simulink model "gm_sobelFilter2024a"  (R2024a)
settings: Solver=FixedStepDiscrete  StartTime=0.0  StopTime=2  FixedStep=1/(R*C)  RelTol=1e-3
undefined symbols (not defined in the file or in its folder): gray, R
libraries: hdlsllib x5, visionhdlio x4, visionsources x2, hdlmdlgenlib x1
(part 2 of 2)

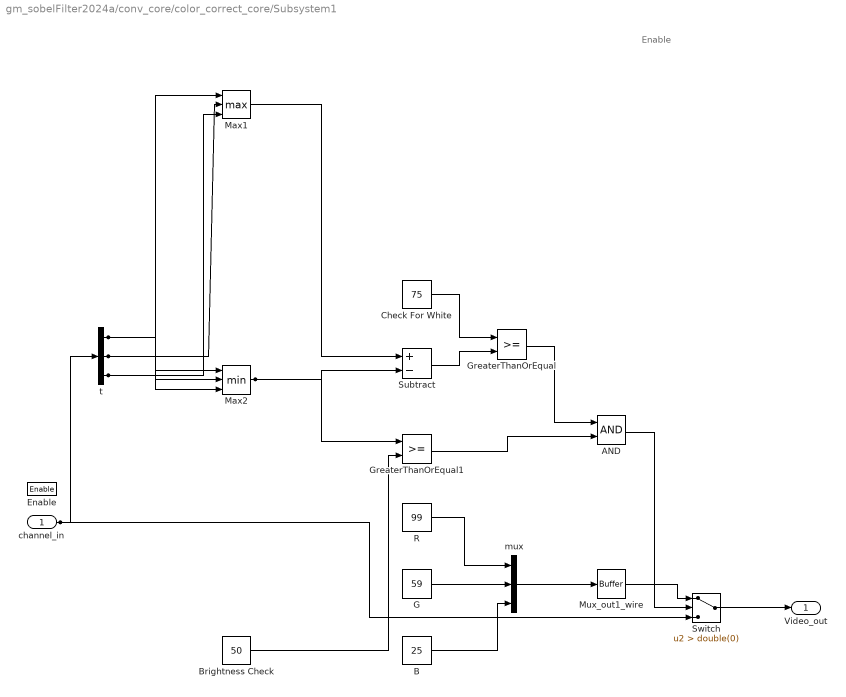
== system gm_sobelFilter2024a/conv_core/color_correct_core/Subsystem1 ==
  note: Enable
  channel_in : Inport  OutDataTypeStr=uint8  PortDimensions=[1 3]  SampleTime=2.77039007092199e-06
  Enable : EnablePort  OutDataTypeStr=boolean
  AND : Logic  AllPortsSameDT=off  OutDataTypeStr=boolean  SampleTime=2.77039007092199e-06
  B : Constant  Value=25  OutDataTypeStr=uint8  SampleTime=2.77039007092199e-06
  Brightness Check : Constant  Value=50  OutDataTypeStr=uint8  SampleTime=2.77039007092199e-06
  Check For White : Constant  Value=75  OutDataTypeStr=uint8  SampleTime=2.77039007092199e-06
  G : Constant  Value=59  OutDataTypeStr=uint8  SampleTime=2.77039007092199e-06
  GreaterThanOrEqual : RelationalOperator  OutDataTypeStr=boolean  SampleTime=2.77039007092199e-06  InputSameDT=off
  GreaterThanOrEqual1 : RelationalOperator  OutDataTypeStr=boolean  SampleTime=2.77039007092199e-06  InputSameDT=off
  Max1 : MinMax  Function=max  Inputs=3  OutDataTypeStr=uint8
  Max2 : MinMax  Inputs=3  OutDataTypeStr=uint8
  Mux_out1_wire : hdlmdlgenlib/Buffer
  R : Constant  Value=99  OutDataTypeStr=uint8  SampleTime=2.77039007092199e-06
  Subtract : Sum  Inputs=+-  OutDataTypeStr=fixdt(1, 9, 0)  AccumDataTypeStr=fixdt(1, 9, 0)  SampleTime=2.77039007092199e-06
  Switch : Switch  Criteria=u2 > Threshold  Threshold=double(0)  OutDataTypeStr=uint8  SampleTime=2.77039007092199e-06  SaturateOnIntegerOverflow=off  InputSameDT=off
  mux : Mux  Inputs=3
  t : Demux  Outputs=3
  Video_out : Outport  OutDataTypeStr=uint8  SampleTime=2.77039007092199e-06  InitialOutput=0
  wires:
  channel_in/1 -> Switch/3, t/1
  AND/1 -> Switch/2
  B/1 -> mux/3
  Brightness Check/1 -> GreaterThanOrEqual1/2
  Check For White/1 -> GreaterThanOrEqual/1
  G/1 -> mux/2
  GreaterThanOrEqual/1 -> AND/1
  GreaterThanOrEqual1/1 -> AND/2
  Max1/1 -> Subtract/1
  Max2/1 -> Subtract/2, GreaterThanOrEqual1/1
  mux/1 -> Mux_out1_wire/1
  R/1 -> mux/1
  Subtract/1 -> GreaterThanOrEqual/2
  Switch/1 -> Video_out/1
  t/1 -> Max1/1, Max2/1
  t/2 -> Max1/2, Max2/2
  t/3 -> Max1/3, Max2/3
  Mux_out1_wire/1 -> Switch/1

== system gm_sobelFilter2024a/conv_core/gaussian_conv_core/Subsystem1 ==
  note: Enable
  note: slice out gray
  channel_in : Inport  OutDataTypeStr=uint8  PortDimensions=1  SampleTime=2.77039007092199e-06
  coeffs : Inport  Port=2  OutDataTypeStr=fixdt(1, 16, 12)  PortDimensions=[9]  SampleTime=2.77039007092199e-06
  Enable : EnablePort  OutDataTypeStr=boolean
  Delay1 : Delay  DelayLength=double(1)  InitialCondition=0
  Delay2 : Delay  DelayLength=double(1)  InitialCondition=0
  Product : Product  Inputs=**  OutDataTypeStr=fixdt(1, 24, 12)  SaturateOnIntegerOverflow=on  SampleTime=2.77039007092199e-06
  Sum of Elements : Sum  Inputs=+  OutDataTypeStr=uint8  SaturateOnIntegerOverflow=on
  mux : Mux  Inputs=9
  slicer : Subsystem
  Video_out : Outport  OutDataTypeStr=uint8  SampleTime=2.77039007092199e-06  InitialOutput=0
  wires:
  channel_in/1 -> slicer/1(channel_in)
  coeffs/1 -> Product/1
  Delay1/1 -> Sum of Elements/1
  Delay2/1 -> Video_out/1
  mux/1 -> Product/2
  Product/1 -> Delay1/1
  Sum of Elements/1 -> Delay2/1
  slicer/1(out_1) -> mux/1
  slicer/2(out_2) -> mux/2
  slicer/3(out_3) -> mux/3
  slicer/4(out_4) -> mux/4
  slicer/5(out_5) -> mux/5
  slicer/6(out_6) -> mux/6
  slicer/7(out_7) -> mux/7
  slicer/8(out_8) -> mux/8
  slicer/9(out_9) -> mux/9

== system gm_sobelFilter2024a/conv_core/just_gray_core/Subsystem1 ==
  note: Enable
  note: Grayscale = (R * 0.25) + (G * 0.5) + (B * 0.0625)
  note: slice out gray
  channel_in : Inport  OutDataTypeStr=uint8  PortDimensions=[1 3]  SampleTime=2.77039007092199e-06
  Enable : EnablePort  OutDataTypeStr=boolean
  Shift Arithmetic3 : ArithShift  BitShiftNumber=double(1)  BinPtShiftNumber=double(0)
  Shift Arithmetic4 : ArithShift  BitShiftNumber=double(2)  BinPtShiftNumber=double(0)
  Shift Arithmetic5 : ArithShift  BitShiftNumber=double(4)  BinPtShiftNumber=double(0)
  Sum_stage2 : Sum  OutDataTypeStr=fixdt(0, 9, 0)  AccumDataTypeStr=uint8  SampleTime=2.77039007092199e-06
  Sum_stage3 : Sum  OutDataTypeStr=uint8  AccumDataTypeStr=uint8  SampleTime=2.77039007092199e-06
  t : Demux  Outputs=3
  Video_out : Outport  OutDataTypeStr=uint8  SampleTime=2.77039007092199e-06  InitialOutput=0
  wires:
  channel_in/1 -> t/1
  Shift Arithmetic3/1 -> Sum_stage2/2
  Shift Arithmetic4/1 -> Sum_stage2/1
  Shift Arithmetic5/1 -> Sum_stage3/2
  Sum_stage3/1 -> Video_out/1
  t/1 -> Shift Arithmetic4/1
  t/2 -> Shift Arithmetic3/1
  t/3 -> Shift Arithmetic5/1
  Sum_stage2/1 -> Sum_stage3/1

== system gm_sobelFilter2024a/conv_core/normalize image/Subsystem1 ==
  note: Enable
  note: Normalize Image (Assuming Max is 115)
  channel_in : Inport  OutDataTypeStr=uint8  PortDimensions=1  SampleTime=2.77039007092199e-06
  Enable : EnablePort  OutDataTypeStr=boolean
  Delay2 : Delay  DelayLength=double(4)  InitialCondition=0
  GreaterThanOrEqual : RelationalOperator  OutDataTypeStr=boolean  SampleTime=2.77039007092199e-06  InputSameDT=off
  Max1 : Constant  Value=115  OutDataTypeStr=uint8  SampleTime=2.77039007092199e-06
  Max2 : Constant  Value=0  OutDataTypeStr=uint8  SampleTime=2.77039007092199e-06
  Switch1 : Switch  Criteria=u2 > Threshold  Threshold=double(0)  OutDataTypeStr=uint8  SampleTime=2.77039007092199e-06  SaturateOnIntegerOverflow=off  InputSameDT=off
  Video_out : Outport  OutDataTypeStr=uint8  SampleTime=2.77039007092199e-06  InitialOutput=0
  wires:
  channel_in/1 -> Switch1/1, GreaterThanOrEqual/1
  Delay2/1 -> Video_out/1
  GreaterThanOrEqual/1 -> Switch1/2
  Max1/1 -> GreaterThanOrEqual/2
  Max2/1 -> Switch1/3
  Switch1/1 -> Delay2/1

== system gm_sobelFilter2024a/conv_core/sobel_horz_conv_core/Subsystem1 ==
  note: Enable
  note: slice out gray
  channel_in : Inport  OutDataTypeStr=uint8  PortDimensions=1  SampleTime=2.77039007092199e-06
  coeffs : Inport  Port=2  OutDataTypeStr=fixdt(1, 16, 12)  PortDimensions=[9]  SampleTime=2.77039007092199e-06
  Enable : EnablePort  OutDataTypeStr=boolean
  Delay1 : Delay  DelayLength=double(1)  InitialCondition=0
  Delay2 : Delay  DelayLength=double(1)  InitialCondition=0
  Product : Product  Inputs=**  OutDataTypeStr=fixdt(1, 24, 12)  SaturateOnIntegerOverflow=on  SampleTime=2.77039007092199e-06
  Sum of Elements : Sum  Inputs=+  OutDataTypeStr=uint8  SaturateOnIntegerOverflow=on
  mux : Mux  Inputs=9
  slicer : Subsystem
  Video_out : Outport  OutDataTypeStr=uint8  SampleTime=2.77039007092199e-06  InitialOutput=0
  wires:
  channel_in/1 -> slicer/1(channel_in)
  coeffs/1 -> Product/1
  Delay1/1 -> Sum of Elements/1
  Delay2/1 -> Video_out/1
  mux/1 -> Product/2
  Product/1 -> Delay1/1
  Sum of Elements/1 -> Delay2/1
  slicer/1(out_1) -> mux/1
  slicer/2(out_2) -> mux/2
  slicer/3(out_3) -> mux/3
  slicer/4(out_4) -> mux/4
  slicer/5(out_5) -> mux/5
  slicer/6(out_6) -> mux/6
  slicer/7(out_7) -> mux/7
  slicer/8(out_8) -> mux/8
  slicer/9(out_9) -> mux/9

== system gm_sobelFilter2024a/conv_core/sobel_horz_conv_core_alt/Subsystem1 ==
  note: Enable
  note: slice out gray
  channel_in : Inport  OutDataTypeStr=uint8  PortDimensions=1  SampleTime=2.77039007092199e-06
  coeffs : Inport  Port=2  OutDataTypeStr=fixdt(1, 16, 12)  PortDimensions=[9]  SampleTime=2.77039007092199e-06
  Enable : EnablePort  OutDataTypeStr=boolean
  Delay1 : Delay  DelayLength=double(1)  InitialCondition=0
  Delay2 : Delay  DelayLength=double(1)  InitialCondition=0
  Product : Product  Inputs=**  OutDataTypeStr=fixdt(1, 24, 12)  SaturateOnIntegerOverflow=on  SampleTime=2.77039007092199e-06
  Sum of Elements : Sum  Inputs=+  OutDataTypeStr=uint8  SaturateOnIntegerOverflow=on
  mux : Mux  Inputs=9
  slicer : Subsystem
  Video_out : Outport  OutDataTypeStr=uint8  SampleTime=2.77039007092199e-06  InitialOutput=0
  wires:
  channel_in/1 -> slicer/1(channel_in)
  coeffs/1 -> Product/1
  Delay1/1 -> Sum of Elements/1
  Delay2/1 -> Video_out/1
  mux/1 -> Product/2
  Product/1 -> Delay1/1
  Sum of Elements/1 -> Delay2/1
  slicer/1(out_1) -> mux/1
  slicer/2(out_2) -> mux/2
  slicer/3(out_3) -> mux/3
  slicer/4(out_4) -> mux/4
  slicer/5(out_5) -> mux/5
  slicer/6(out_6) -> mux/6
  slicer/7(out_7) -> mux/7
  slicer/8(out_8) -> mux/8
  slicer/9(out_9) -> mux/9

== system gm_sobelFilter2024a/conv_core/sobel_vert_conv_core/Subsystem1 ==
  note: Enable
  note: slice out gray
  channel_in : Inport  OutDataTypeStr=uint8  PortDimensions=1  SampleTime=2.77039007092199e-06
  coeffs : Inport  Port=2  OutDataTypeStr=fixdt(1, 16, 12)  PortDimensions=[9]  SampleTime=2.77039007092199e-06
  Enable : EnablePort  OutDataTypeStr=boolean
  Delay1 : Delay  DelayLength=double(1)  InitialCondition=0
  Delay2 : Delay  DelayLength=double(1)  InitialCondition=0
  Product : Product  Inputs=**  OutDataTypeStr=fixdt(1, 24, 12)  SaturateOnIntegerOverflow=on  SampleTime=2.77039007092199e-06
  Sum of Elements : Sum  Inputs=+  OutDataTypeStr=uint8  SaturateOnIntegerOverflow=on
  mux : Mux  Inputs=9
  slicer : Subsystem
  Video_out : Outport  OutDataTypeStr=uint8  SampleTime=2.77039007092199e-06  InitialOutput=0
  wires:
  channel_in/1 -> slicer/1(channel_in)
  coeffs/1 -> Product/1
  Delay1/1 -> Sum of Elements/1
  Delay2/1 -> Video_out/1
  mux/1 -> Product/2
  Product/1 -> Delay1/1
  Sum of Elements/1 -> Delay2/1
  slicer/1(out_1) -> mux/1
  slicer/2(out_2) -> mux/2
  slicer/3(out_3) -> mux/3
  slicer/4(out_4) -> mux/4
  slicer/5(out_5) -> mux/5
  slicer/6(out_6) -> mux/6
  slicer/7(out_7) -> mux/7
  slicer/8(out_8) -> mux/8
  slicer/9(out_9) -> mux/9

== system gm_sobelFilter2024a/conv_core/sobel_vert_conv_core_alt/Subsystem1 ==
  note: Enable
  note: slice out gray
  channel_in : Inport  OutDataTypeStr=uint8  PortDimensions=1  SampleTime=2.77039007092199e-06
  coeffs : Inport  Port=2  OutDataTypeStr=fixdt(1, 16, 12)  PortDimensions=[9]  SampleTime=2.77039007092199e-06
  Enable : EnablePort  OutDataTypeStr=boolean
  Delay1 : Delay  DelayLength=double(1)  InitialCondition=0
  Delay2 : Delay  DelayLength=double(1)  InitialCondition=0
  Product : Product  Inputs=**  OutDataTypeStr=fixdt(1, 24, 12)  SaturateOnIntegerOverflow=on  SampleTime=2.77039007092199e-06
  Sum of Elements : Sum  Inputs=+  OutDataTypeStr=uint8  SaturateOnIntegerOverflow=on
  mux : Mux  Inputs=9
  slicer : Subsystem
  Video_out : Outport  OutDataTypeStr=uint8  SampleTime=2.77039007092199e-06  InitialOutput=0
  wires:
  channel_in/1 -> slicer/1(channel_in)
  coeffs/1 -> Product/1
  Delay1/1 -> Sum of Elements/1
  Delay2/1 -> Video_out/1
  mux/1 -> Product/2
  Product/1 -> Delay1/1
  Sum of Elements/1 -> Delay2/1
  slicer/1(out_1) -> mux/1
  slicer/2(out_2) -> mux/2
  slicer/3(out_3) -> mux/3
  slicer/4(out_4) -> mux/4
  slicer/5(out_5) -> mux/5
  slicer/6(out_6) -> mux/6
  slicer/7(out_7) -> mux/7
  slicer/8(out_8) -> mux/8
  slicer/9(out_9) -> mux/9

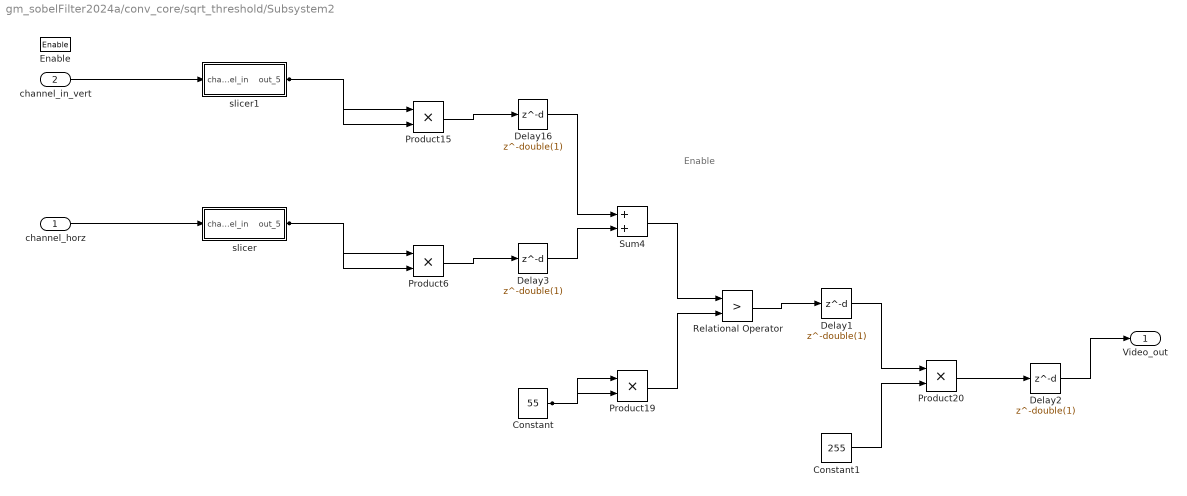
== system gm_sobelFilter2024a/conv_core/sqrt_threshold/Subsystem2 ==
  note: Enable
  channel_horz : Inport  OutDataTypeStr=uint8  PortDimensions=1  SampleTime=2.77039007092199e-06
  channel_in_vert : Inport  Port=2  OutDataTypeStr=uint8  PortDimensions=1  SampleTime=2.77039007092199e-06
  Enable : EnablePort  OutDataTypeStr=boolean
  Constant : Constant  Value=55  OutDataTypeStr=uint8  SampleTime=2.77039007092199e-06
  Constant1 : Constant  Value=255  OutDataTypeStr=uint8  SampleTime=2.77039007092199e-06
  Delay{1..3,16} (4 alike) : Delay  DelayLength=double(1)  InitialCondition=0
  Product15 : Product  Inputs=**  OutDataTypeStr=uint16  SaturateOnIntegerOverflow=on  SampleTime=2.77039007092199e-06
  Product19 : Product  Inputs=**  OutDataTypeStr=uint16  SaturateOnIntegerOverflow=on  SampleTime=2.77039007092199e-06
  Product20 : Product  Inputs=**  OutDataTypeStr=uint8  SaturateOnIntegerOverflow=on  SampleTime=2.77039007092199e-06
  Product6 : Product  Inputs=**  OutDataTypeStr=uint16  SaturateOnIntegerOverflow=on  SampleTime=2.77039007092199e-06
  Relational Operator : RelationalOperator  Operator=>  OutDataTypeStr=boolean  SampleTime=2.77039007092199e-06  InputSameDT=off
  Sum4 : Sum  OutDataTypeStr=fixdt(0, 17, 0)  AccumDataTypeStr=fixdt(0, 17, 0)  SampleTime=2.77039007092199e-06
  slicer : Subsystem
  slicer1 : Subsystem
  Video_out : Outport  OutDataTypeStr=uint8  SampleTime=2.77039007092199e-06  InitialOutput=0
  wires:
  channel_horz/1 -> slicer/1(channel_in)
  channel_in_vert/1 -> slicer1/1(channel_in)
  Constant/1 -> Product19/2, Product19/1
  Constant1/1 -> Product20/2
  Delay1/1 -> Product20/1
  Delay16/1 -> Sum4/1
  Delay2/1 -> Video_out/1
  Delay3/1 -> Sum4/2
  Product15/1 -> Delay16/1
  Product19/1 -> Relational Operator/2
  Product20/1 -> Delay2/1
  Product6/1 -> Delay3/1
  Relational Operator/1 -> Delay1/1
  Sum4/1 -> Relational Operator/1
  slicer/1(out_5) -> Product6/2, Product6/1
  slicer1/1(out_5) -> Product15/2, Product15/1

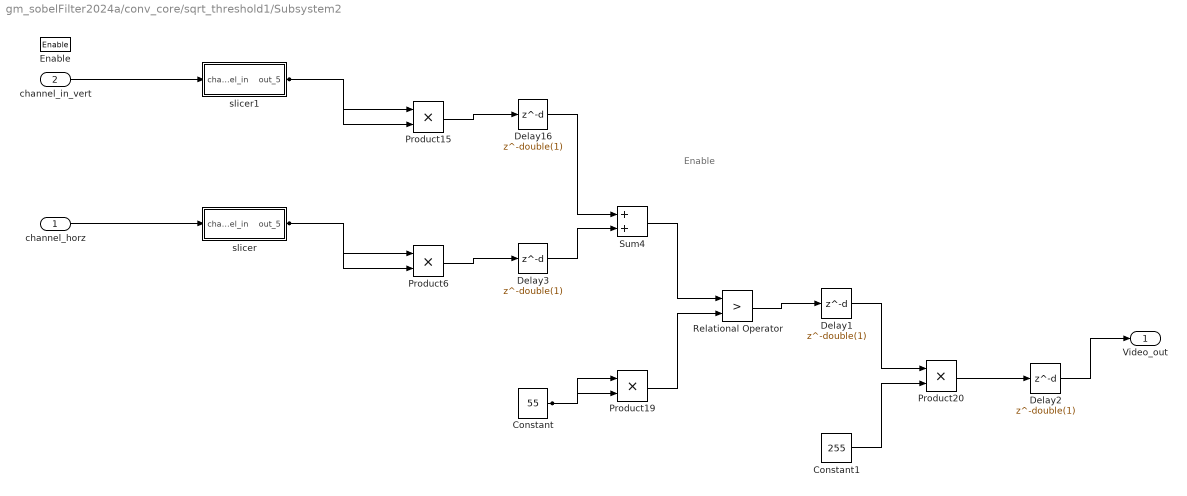
== system gm_sobelFilter2024a/conv_core/sqrt_threshold1/Subsystem2 ==
  note: Enable
  channel_horz : Inport  OutDataTypeStr=uint8  PortDimensions=1  SampleTime=2.77039007092199e-06
  channel_in_vert : Inport  Port=2  OutDataTypeStr=uint8  PortDimensions=1  SampleTime=2.77039007092199e-06
  Enable : EnablePort  OutDataTypeStr=boolean
  Constant : Constant  Value=55  OutDataTypeStr=uint8  SampleTime=2.77039007092199e-06
  Constant1 : Constant  Value=255  OutDataTypeStr=uint8  SampleTime=2.77039007092199e-06
  Delay{1..3,16} (4 alike) : Delay  DelayLength=double(1)  InitialCondition=0
  Product15 : Product  Inputs=**  OutDataTypeStr=uint16  SaturateOnIntegerOverflow=on  SampleTime=2.77039007092199e-06
  Product19 : Product  Inputs=**  OutDataTypeStr=uint16  SaturateOnIntegerOverflow=on  SampleTime=2.77039007092199e-06
  Product20 : Product  Inputs=**  OutDataTypeStr=uint8  SaturateOnIntegerOverflow=on  SampleTime=2.77039007092199e-06
  Product6 : Product  Inputs=**  OutDataTypeStr=uint16  SaturateOnIntegerOverflow=on  SampleTime=2.77039007092199e-06
  Relational Operator : RelationalOperator  Operator=>  OutDataTypeStr=boolean  SampleTime=2.77039007092199e-06  InputSameDT=off
  Sum4 : Sum  OutDataTypeStr=fixdt(0, 17, 0)  AccumDataTypeStr=fixdt(0, 17, 0)  SampleTime=2.77039007092199e-06
  slicer : Subsystem
  slicer1 : Subsystem
  Video_out : Outport  OutDataTypeStr=uint8  SampleTime=2.77039007092199e-06  InitialOutput=0
  wires:
  slicer1/1(out_5) -> Product15/1, Product15/2
  slicer/1(out_5) -> Product6/1, Product6/2
  Sum4/1 -> Relational Operator/1
  Relational Operator/1 -> Delay1/1
  Product6/1 -> Delay3/1
  Product20/1 -> Delay2/1
  Product19/1 -> Relational Operator/2
  Product15/1 -> Delay16/1
  Delay3/1 -> Sum4/2
  Delay2/1 -> Video_out/1
  Delay16/1 -> Sum4/1
  Delay1/1 -> Product20/1
  Constant1/1 -> Product20/2
  Constant/1 -> Product19/1, Product19/2
  channel_in_vert/1 -> slicer1/1(channel_in)
  channel_horz/1 -> slicer/1(channel_in)

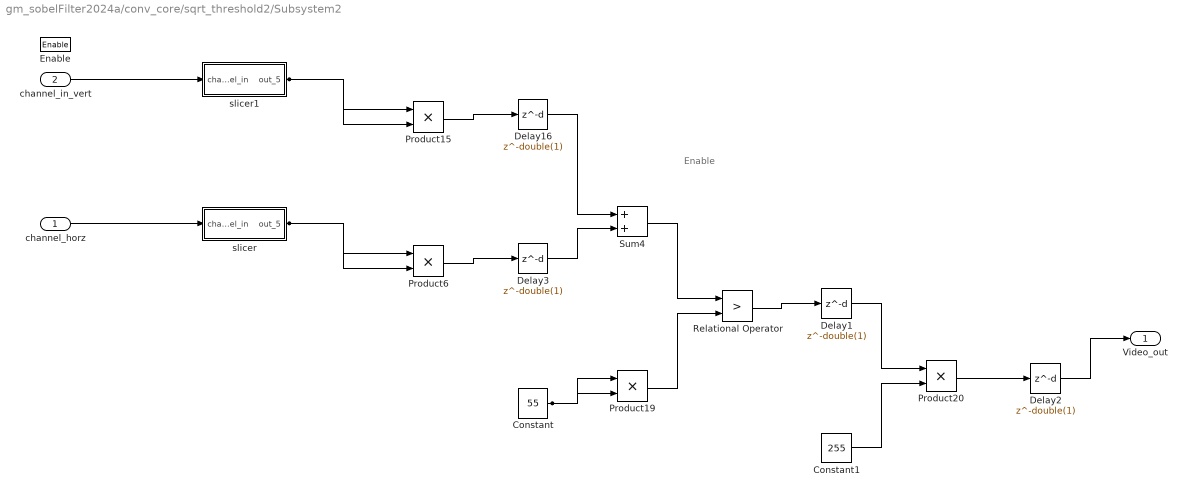
== system gm_sobelFilter2024a/conv_core/sqrt_threshold2/Subsystem2 ==
  note: Enable
  channel_horz : Inport  OutDataTypeStr=uint8  PortDimensions=1  SampleTime=2.77039007092199e-06
  channel_in_vert : Inport  Port=2  OutDataTypeStr=uint8  PortDimensions=1  SampleTime=2.77039007092199e-06
  Enable : EnablePort  OutDataTypeStr=boolean
  Constant : Constant  Value=55  OutDataTypeStr=uint8  SampleTime=2.77039007092199e-06
  Constant1 : Constant  Value=255  OutDataTypeStr=uint8  SampleTime=2.77039007092199e-06
  Delay{1..3,16} (4 alike) : Delay  DelayLength=double(1)  InitialCondition=0
  Product15 : Product  Inputs=**  OutDataTypeStr=uint16  SaturateOnIntegerOverflow=on  SampleTime=2.77039007092199e-06
  Product19 : Product  Inputs=**  OutDataTypeStr=uint16  SaturateOnIntegerOverflow=on  SampleTime=2.77039007092199e-06
  Product20 : Product  Inputs=**  OutDataTypeStr=uint8  SaturateOnIntegerOverflow=on  SampleTime=2.77039007092199e-06
  Product6 : Product  Inputs=**  OutDataTypeStr=uint16  SaturateOnIntegerOverflow=on  SampleTime=2.77039007092199e-06
  Relational Operator : RelationalOperator  Operator=>  OutDataTypeStr=boolean  SampleTime=2.77039007092199e-06  InputSameDT=off
  Sum4 : Sum  OutDataTypeStr=fixdt(0, 17, 0)  AccumDataTypeStr=fixdt(0, 17, 0)  SampleTime=2.77039007092199e-06
  slicer : Subsystem
  slicer1 : Subsystem
  Video_out : Outport  OutDataTypeStr=uint8  SampleTime=2.77039007092199e-06  InitialOutput=0
  wires:
  slicer1/1(out_5) -> Product15/1, Product15/2
  slicer/1(out_5) -> Product6/1, Product6/2
  Sum4/1 -> Relational Operator/1
  Relational Operator/1 -> Delay1/1
  Product6/1 -> Delay3/1
  Product20/1 -> Delay2/1
  Product19/1 -> Relational Operator/2
  Product15/1 -> Delay16/1
  Delay3/1 -> Sum4/2
  Delay2/1 -> Video_out/1
  Delay16/1 -> Sum4/1
  Delay1/1 -> Product20/1
  Constant1/1 -> Product20/2
  Constant/1 -> Product19/1, Product19/2
  channel_in_vert/1 -> slicer1/1(channel_in)
  channel_horz/1 -> slicer/1(channel_in)

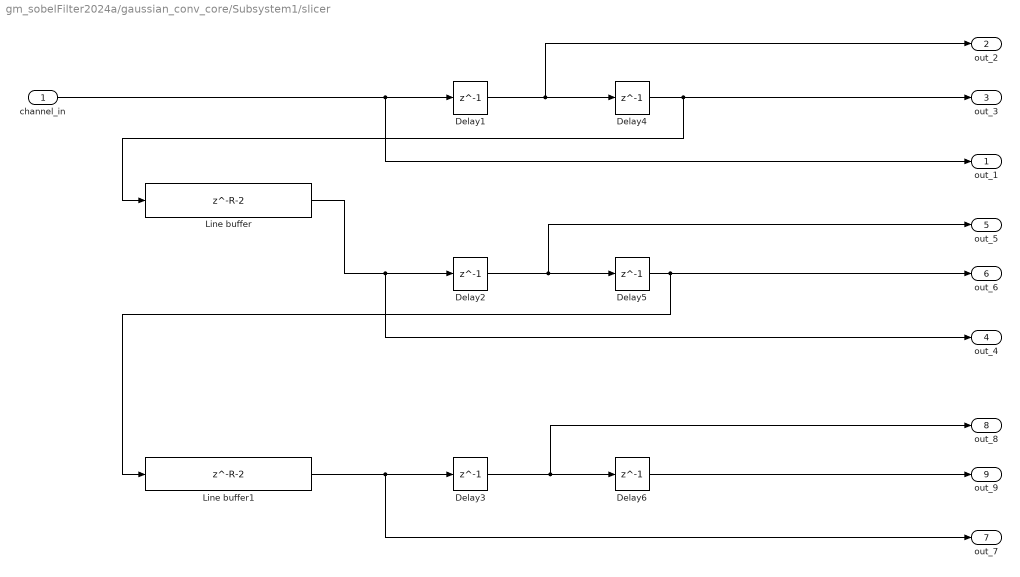
== system gm_sobelFilter2024a/gaussian_conv_core/Subsystem1/slicer ==
  channel_in : Inport
  Delay{1..6} (6 alike) : Delay  DelayLength=1  InitialCondition=0
  Line buffer : Delay  DelayLength=R-2  InitialCondition=0
  Line buffer1 : Delay  DelayLength=R-2  InitialCondition=0
  out_1 : Outport  VectorParamsAs1DForOutWhenUnconnected=off
  out_2 : Outport  Port=2  VectorParamsAs1DForOutWhenUnconnected=off
  out_3 : Outport  Port=3  VectorParamsAs1DForOutWhenUnconnected=off
  out_4 : Outport  Port=4  VectorParamsAs1DForOutWhenUnconnected=off
  out_5 : Outport  Port=5  VectorParamsAs1DForOutWhenUnconnected=off
  out_6 : Outport  Port=6  VectorParamsAs1DForOutWhenUnconnected=off
  out_7 : Outport  Port=7  VectorParamsAs1DForOutWhenUnconnected=off
  out_8 : Outport  Port=8  VectorParamsAs1DForOutWhenUnconnected=off
  out_9 : Outport  Port=9  VectorParamsAs1DForOutWhenUnconnected=off
  wires:
  Delay2/1 -> Delay5/1, out_5/1
  Line buffer1/1 -> Delay3/1, out_7/1
  Line buffer/1 -> Delay2/1, out_4/1
  Delay6/1 -> out_9/1
  Delay5/1 -> out_6/1, Line buffer1/1
  Delay3/1 -> Delay6/1, out_8/1
  Delay1/1 -> Delay4/1, out_2/1
  channel_in/1 -> Delay1/1, out_1/1
  Delay4/1 -> out_3/1, Line buffer/1

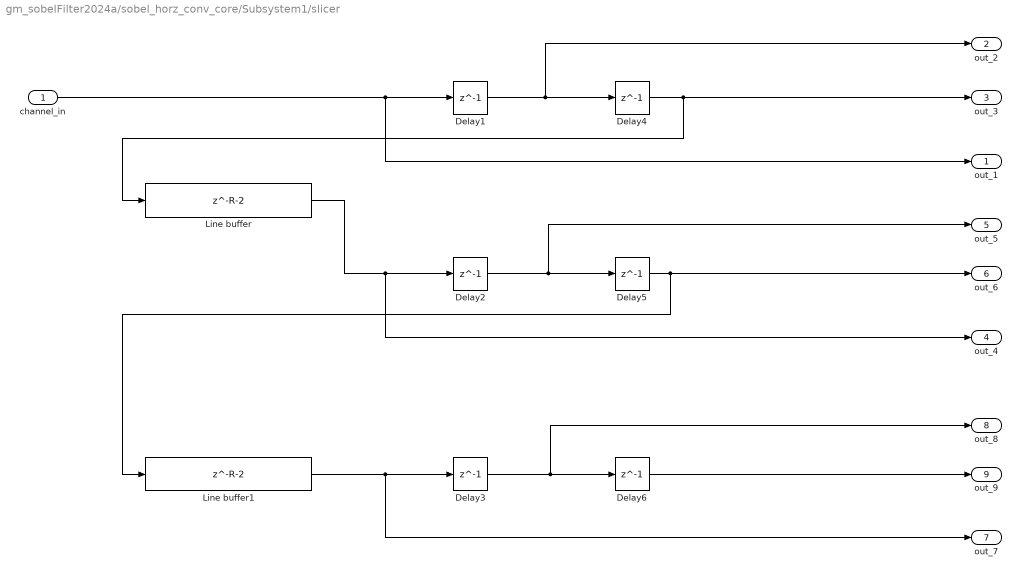
== system gm_sobelFilter2024a/sobel_horz_conv_core/Subsystem1/slicer ==
  channel_in : Inport
  Delay{1..6} (6 alike) : Delay  DelayLength=1  InitialCondition=0
  Line buffer : Delay  DelayLength=R-2  InitialCondition=0
  Line buffer1 : Delay  DelayLength=R-2  InitialCondition=0
  out_1 : Outport  VectorParamsAs1DForOutWhenUnconnected=off
  out_2 : Outport  Port=2  VectorParamsAs1DForOutWhenUnconnected=off
  out_3 : Outport  Port=3  VectorParamsAs1DForOutWhenUnconnected=off
  out_4 : Outport  Port=4  VectorParamsAs1DForOutWhenUnconnected=off
  out_5 : Outport  Port=5  VectorParamsAs1DForOutWhenUnconnected=off
  out_6 : Outport  Port=6  VectorParamsAs1DForOutWhenUnconnected=off
  out_7 : Outport  Port=7  VectorParamsAs1DForOutWhenUnconnected=off
  out_8 : Outport  Port=8  VectorParamsAs1DForOutWhenUnconnected=off
  out_9 : Outport  Port=9  VectorParamsAs1DForOutWhenUnconnected=off
  wires:
  Delay2/1 -> Delay5/1, out_5/1
  Line buffer1/1 -> Delay3/1, out_7/1
  Line buffer/1 -> Delay2/1, out_4/1
  Delay6/1 -> out_9/1
  Delay5/1 -> out_6/1, Line buffer1/1
  Delay3/1 -> Delay6/1, out_8/1
  Delay1/1 -> Delay4/1, out_2/1
  channel_in/1 -> Delay1/1, out_1/1
  Delay4/1 -> out_3/1, Line buffer/1

== system gm_sobelFilter2024a/sobel_horz_conv_core_alt/Subsystem1/slicer ==
  channel_in : Inport
  Delay{1..6} (6 alike) : Delay  DelayLength=1  InitialCondition=0
  Line buffer : Delay  DelayLength=R-2  InitialCondition=0
  Line buffer1 : Delay  DelayLength=R-2  InitialCondition=0
  out_1 : Outport  VectorParamsAs1DForOutWhenUnconnected=off
  out_2 : Outport  Port=2  VectorParamsAs1DForOutWhenUnconnected=off
  out_3 : Outport  Port=3  VectorParamsAs1DForOutWhenUnconnected=off
  out_4 : Outport  Port=4  VectorParamsAs1DForOutWhenUnconnected=off
  out_5 : Outport  Port=5  VectorParamsAs1DForOutWhenUnconnected=off
  out_6 : Outport  Port=6  VectorParamsAs1DForOutWhenUnconnected=off
  out_7 : Outport  Port=7  VectorParamsAs1DForOutWhenUnconnected=off
  out_8 : Outport  Port=8  VectorParamsAs1DForOutWhenUnconnected=off
  out_9 : Outport  Port=9  VectorParamsAs1DForOutWhenUnconnected=off
  wires:
  Delay2/1 -> Delay5/1, out_5/1
  Line buffer1/1 -> Delay3/1, out_7/1
  Line buffer/1 -> Delay2/1, out_4/1
  Delay6/1 -> out_9/1
  Delay5/1 -> out_6/1, Line buffer1/1
  Delay3/1 -> Delay6/1, out_8/1
  Delay1/1 -> Delay4/1, out_2/1
  channel_in/1 -> Delay1/1, out_1/1
  Delay4/1 -> out_3/1, Line buffer/1

== system gm_sobelFilter2024a/sobel_vert_conv_core/Subsystem1/slicer ==
  channel_in : Inport
  Delay{1..6} (6 alike) : Delay  DelayLength=1  InitialCondition=0
  Line buffer : Delay  DelayLength=R-2  InitialCondition=0
  Line buffer1 : Delay  DelayLength=R-2  InitialCondition=0
  out_1 : Outport  VectorParamsAs1DForOutWhenUnconnected=off
  out_2 : Outport  Port=2  VectorParamsAs1DForOutWhenUnconnected=off
  out_3 : Outport  Port=3  VectorParamsAs1DForOutWhenUnconnected=off
  out_4 : Outport  Port=4  VectorParamsAs1DForOutWhenUnconnected=off
  out_5 : Outport  Port=5  VectorParamsAs1DForOutWhenUnconnected=off
  out_6 : Outport  Port=6  VectorParamsAs1DForOutWhenUnconnected=off
  out_7 : Outport  Port=7  VectorParamsAs1DForOutWhenUnconnected=off
  out_8 : Outport  Port=8  VectorParamsAs1DForOutWhenUnconnected=off
  out_9 : Outport  Port=9  VectorParamsAs1DForOutWhenUnconnected=off
  wires:
  Delay2/1 -> Delay5/1, out_5/1
  Line buffer1/1 -> Delay3/1, out_7/1
  Line buffer/1 -> Delay2/1, out_4/1
  Delay6/1 -> out_9/1
  Delay5/1 -> out_6/1, Line buffer1/1
  Delay3/1 -> Delay6/1, out_8/1
  Delay1/1 -> Delay4/1, out_2/1
  channel_in/1 -> Delay1/1, out_1/1
  Delay4/1 -> out_3/1, Line buffer/1

== system gm_sobelFilter2024a/sobel_vert_conv_core_alt/Subsystem1/slicer ==
  channel_in : Inport
  Delay{1..6} (6 alike) : Delay  DelayLength=1  InitialCondition=0
  Line buffer : Delay  DelayLength=R-2  InitialCondition=0
  Line buffer1 : Delay  DelayLength=R-2  InitialCondition=0
  out_1 : Outport  VectorParamsAs1DForOutWhenUnconnected=off
  out_2 : Outport  Port=2  VectorParamsAs1DForOutWhenUnconnected=off
  out_3 : Outport  Port=3  VectorParamsAs1DForOutWhenUnconnected=off
  out_4 : Outport  Port=4  VectorParamsAs1DForOutWhenUnconnected=off
  out_5 : Outport  Port=5  VectorParamsAs1DForOutWhenUnconnected=off
  out_6 : Outport  Port=6  VectorParamsAs1DForOutWhenUnconnected=off
  out_7 : Outport  Port=7  VectorParamsAs1DForOutWhenUnconnected=off
  out_8 : Outport  Port=8  VectorParamsAs1DForOutWhenUnconnected=off
  out_9 : Outport  Port=9  VectorParamsAs1DForOutWhenUnconnected=off
  wires:
  Delay2/1 -> Delay5/1, out_5/1
  Line buffer1/1 -> Delay3/1, out_7/1
  Line buffer/1 -> Delay2/1, out_4/1
  Delay6/1 -> out_9/1
  Delay5/1 -> out_6/1, Line buffer1/1
  Delay3/1 -> Delay6/1, out_8/1
  Delay1/1 -> Delay4/1, out_2/1
  channel_in/1 -> Delay1/1, out_1/1
  Delay4/1 -> out_3/1, Line buffer/1

== system gm_sobelFilter2024a/sqrt_threshold/Subsystem2/slicer ==
  channel_in : Inport
  Delay{1..6} (6 alike) : Delay  DelayLength=1  InitialCondition=0
  Line buffer : Delay  DelayLength=R-2  InitialCondition=0
  Line buffer1 : Delay  DelayLength=R-2  InitialCondition=0
  out_1 : Outport  VectorParamsAs1DForOutWhenUnconnected=off
  out_2 : Outport  Port=2  VectorParamsAs1DForOutWhenUnconnected=off
  out_3 : Outport  Port=3  VectorParamsAs1DForOutWhenUnconnected=off
  out_4 : Outport  Port=4  VectorParamsAs1DForOutWhenUnconnected=off
  out_5 : Outport  Port=5  VectorParamsAs1DForOutWhenUnconnected=off
  out_6 : Outport  Port=6  VectorParamsAs1DForOutWhenUnconnected=off
  out_7 : Outport  Port=7  VectorParamsAs1DForOutWhenUnconnected=off
  out_8 : Outport  Port=8  VectorParamsAs1DForOutWhenUnconnected=off
  out_9 : Outport  Port=9  VectorParamsAs1DForOutWhenUnconnected=off
  wires:
  Delay2/1 -> Delay5/1, out_5/1
  Line buffer1/1 -> Delay3/1, out_7/1
  Line buffer/1 -> Delay2/1, out_4/1
  Delay6/1 -> out_9/1
  Delay5/1 -> out_6/1, Line buffer1/1
  Delay3/1 -> Delay6/1, out_8/1
  Delay1/1 -> Delay4/1, out_2/1
  channel_in/1 -> Delay1/1, out_1/1
  Delay4/1 -> out_3/1, Line buffer/1

== system gm_sobelFilter2024a/sqrt_threshold/Subsystem2/slicer1 ==
  channel_in : Inport
  Delay{1..6} (6 alike) : Delay  DelayLength=1  InitialCondition=0
  Line buffer : Delay  DelayLength=R-2  InitialCondition=0
  Line buffer1 : Delay  DelayLength=R-2  InitialCondition=0
  out_1 : Outport  VectorParamsAs1DForOutWhenUnconnected=off
  out_2 : Outport  Port=2  VectorParamsAs1DForOutWhenUnconnected=off
  out_3 : Outport  Port=3  VectorParamsAs1DForOutWhenUnconnected=off
  out_4 : Outport  Port=4  VectorParamsAs1DForOutWhenUnconnected=off
  out_5 : Outport  Port=5  VectorParamsAs1DForOutWhenUnconnected=off
  out_6 : Outport  Port=6  VectorParamsAs1DForOutWhenUnconnected=off
  out_7 : Outport  Port=7  VectorParamsAs1DForOutWhenUnconnected=off
  out_8 : Outport  Port=8  VectorParamsAs1DForOutWhenUnconnected=off
  out_9 : Outport  Port=9  VectorParamsAs1DForOutWhenUnconnected=off
  wires:
  Delay2/1 -> Delay5/1, out_5/1
  Line buffer1/1 -> Delay3/1, out_7/1
  Line buffer/1 -> Delay2/1, out_4/1
  Delay6/1 -> out_9/1
  Delay5/1 -> out_6/1, Line buffer1/1
  Delay3/1 -> Delay6/1, out_8/1
  Delay1/1 -> Delay4/1, out_2/1
  channel_in/1 -> Delay1/1, out_1/1
  Delay4/1 -> out_3/1, Line buffer/1

== system gm_sobelFilter2024a/sqrt_threshold1/Subsystem2/slicer ==
  channel_in : Inport
  Delay{1..6} (6 alike) : Delay  DelayLength=1  InitialCondition=0
  Line buffer : Delay  DelayLength=R-2  InitialCondition=0
  Line buffer1 : Delay  DelayLength=R-2  InitialCondition=0
  out_1 : Outport  VectorParamsAs1DForOutWhenUnconnected=off
  out_2 : Outport  Port=2  VectorParamsAs1DForOutWhenUnconnected=off
  out_3 : Outport  Port=3  VectorParamsAs1DForOutWhenUnconnected=off
  out_4 : Outport  Port=4  VectorParamsAs1DForOutWhenUnconnected=off
  out_5 : Outport  Port=5  VectorParamsAs1DForOutWhenUnconnected=off
  out_6 : Outport  Port=6  VectorParamsAs1DForOutWhenUnconnected=off
  out_7 : Outport  Port=7  VectorParamsAs1DForOutWhenUnconnected=off
  out_8 : Outport  Port=8  VectorParamsAs1DForOutWhenUnconnected=off
  out_9 : Outport  Port=9  VectorParamsAs1DForOutWhenUnconnected=off
  wires:
  Delay2/1 -> Delay5/1, out_5/1
  Line buffer1/1 -> Delay3/1, out_7/1
  Line buffer/1 -> Delay2/1, out_4/1
  Delay6/1 -> out_9/1
  Delay5/1 -> out_6/1, Line buffer1/1
  Delay3/1 -> Delay6/1, out_8/1
  Delay1/1 -> Delay4/1, out_2/1
  channel_in/1 -> Delay1/1, out_1/1
  Delay4/1 -> out_3/1, Line buffer/1

== system gm_sobelFilter2024a/sqrt_threshold1/Subsystem2/slicer1 ==
  channel_in : Inport
  Delay{1..6} (6 alike) : Delay  DelayLength=1  InitialCondition=0
  Line buffer : Delay  DelayLength=R-2  InitialCondition=0
  Line buffer1 : Delay  DelayLength=R-2  InitialCondition=0
  out_1 : Outport  VectorParamsAs1DForOutWhenUnconnected=off
  out_2 : Outport  Port=2  VectorParamsAs1DForOutWhenUnconnected=off
  out_3 : Outport  Port=3  VectorParamsAs1DForOutWhenUnconnected=off
  out_4 : Outport  Port=4  VectorParamsAs1DForOutWhenUnconnected=off
  out_5 : Outport  Port=5  VectorParamsAs1DForOutWhenUnconnected=off
  out_6 : Outport  Port=6  VectorParamsAs1DForOutWhenUnconnected=off
  out_7 : Outport  Port=7  VectorParamsAs1DForOutWhenUnconnected=off
  out_8 : Outport  Port=8  VectorParamsAs1DForOutWhenUnconnected=off
  out_9 : Outport  Port=9  VectorParamsAs1DForOutWhenUnconnected=off
  wires:
  Delay2/1 -> Delay5/1, out_5/1
  Line buffer1/1 -> Delay3/1, out_7/1
  Line buffer/1 -> Delay2/1, out_4/1
  Delay6/1 -> out_9/1
  Delay5/1 -> out_6/1, Line buffer1/1
  Delay3/1 -> Delay6/1, out_8/1
  Delay1/1 -> Delay4/1, out_2/1
  channel_in/1 -> Delay1/1, out_1/1
  Delay4/1 -> out_3/1, Line buffer/1

== system gm_sobelFilter2024a/sqrt_threshold2/Subsystem2/slicer ==
  channel_in : Inport
  Delay{1..6} (6 alike) : Delay  DelayLength=1  InitialCondition=0
  Line buffer : Delay  DelayLength=R-2  InitialCondition=0
  Line buffer1 : Delay  DelayLength=R-2  InitialCondition=0
  out_1 : Outport  VectorParamsAs1DForOutWhenUnconnected=off
  out_2 : Outport  Port=2  VectorParamsAs1DForOutWhenUnconnected=off
  out_3 : Outport  Port=3  VectorParamsAs1DForOutWhenUnconnected=off
  out_4 : Outport  Port=4  VectorParamsAs1DForOutWhenUnconnected=off
  out_5 : Outport  Port=5  VectorParamsAs1DForOutWhenUnconnected=off
  out_6 : Outport  Port=6  VectorParamsAs1DForOutWhenUnconnected=off
  out_7 : Outport  Port=7  VectorParamsAs1DForOutWhenUnconnected=off
  out_8 : Outport  Port=8  VectorParamsAs1DForOutWhenUnconnected=off
  out_9 : Outport  Port=9  VectorParamsAs1DForOutWhenUnconnected=off
  wires:
  Delay2/1 -> Delay5/1, out_5/1
  Line buffer1/1 -> Delay3/1, out_7/1
  Line buffer/1 -> Delay2/1, out_4/1
  Delay6/1 -> out_9/1
  Delay5/1 -> out_6/1, Line buffer1/1
  Delay3/1 -> Delay6/1, out_8/1
  Delay1/1 -> Delay4/1, out_2/1
  channel_in/1 -> Delay1/1, out_1/1
  Delay4/1 -> out_3/1, Line buffer/1

== system gm_sobelFilter2024a/sqrt_threshold2/Subsystem2/slicer1 ==
  channel_in : Inport
  Delay{1..6} (6 alike) : Delay  DelayLength=1  InitialCondition=0
  Line buffer : Delay  DelayLength=R-2  InitialCondition=0
  Line buffer1 : Delay  DelayLength=R-2  InitialCondition=0
  out_1 : Outport  VectorParamsAs1DForOutWhenUnconnected=off
  out_2 : Outport  Port=2  VectorParamsAs1DForOutWhenUnconnected=off
  out_3 : Outport  Port=3  VectorParamsAs1DForOutWhenUnconnected=off
  out_4 : Outport  Port=4  VectorParamsAs1DForOutWhenUnconnected=off
  out_5 : Outport  Port=5  VectorParamsAs1DForOutWhenUnconnected=off
  out_6 : Outport  Port=6  VectorParamsAs1DForOutWhenUnconnected=off
  out_7 : Outport  Port=7  VectorParamsAs1DForOutWhenUnconnected=off
  out_8 : Outport  Port=8  VectorParamsAs1DForOutWhenUnconnected=off
  out_9 : Outport  Port=9  VectorParamsAs1DForOutWhenUnconnected=off
  wires:
  Delay2/1 -> Delay5/1, out_5/1
  Line buffer1/1 -> Delay3/1, out_7/1
  Line buffer/1 -> Delay2/1, out_4/1
  Delay6/1 -> out_9/1
  Delay5/1 -> out_6/1, Line buffer1/1
  Delay3/1 -> Delay6/1, out_8/1
  Delay1/1 -> Delay4/1, out_2/1
  channel_in/1 -> Delay1/1, out_1/1
  Delay4/1 -> out_3/1, Line buffer/1

== system gm_sobelFilter2024a/conv_core/gaussian_conv_core/Subsystem1/slicer ==
  channel_in : Inport  OutDataTypeStr=uint8  PortDimensions=1  SampleTime=2.77039007092199e-06
  Delay{1..6} (6 alike) : Delay  DelayLength=double(1)  InitialCondition=0
  Line buffer : Delay  DelayLength=double(750)  InitialCondition=0
  Line buffer1 : Delay  DelayLength=double(750)  InitialCondition=0
  out_1 : Outport  SampleTime=2.77039007092199e-06  InitialOutput=0  VectorParamsAs1DForOutWhenUnconnected=off
  out_2 : Outport  Port=2  SampleTime=2.77039007092199e-06  InitialOutput=0  VectorParamsAs1DForOutWhenUnconnected=off
  out_3 : Outport  Port=3  SampleTime=2.77039007092199e-06  InitialOutput=0  VectorParamsAs1DForOutWhenUnconnected=off
  out_4 : Outport  Port=4  SampleTime=2.77039007092199e-06  InitialOutput=0  VectorParamsAs1DForOutWhenUnconnected=off
  out_5 : Outport  Port=5  SampleTime=2.77039007092199e-06  InitialOutput=0  VectorParamsAs1DForOutWhenUnconnected=off
  out_6 : Outport  Port=6  SampleTime=2.77039007092199e-06  InitialOutput=0  VectorParamsAs1DForOutWhenUnconnected=off
  out_7 : Outport  Port=7  SampleTime=2.77039007092199e-06  InitialOutput=0  VectorParamsAs1DForOutWhenUnconnected=off
  out_8 : Outport  Port=8  SampleTime=2.77039007092199e-06  InitialOutput=0  VectorParamsAs1DForOutWhenUnconnected=off
  out_9 : Outport  Port=9  SampleTime=2.77039007092199e-06  InitialOutput=0  VectorParamsAs1DForOutWhenUnconnected=off
  wires:
  channel_in/1 -> Delay1/1, out_1/1
  Delay1/1 -> Delay4/1, out_2/1
  Delay2/1 -> Delay5/1, out_5/1
  Delay3/1 -> Delay6/1, out_8/1
  Delay4/1 -> Line buffer/1, out_3/1
  Delay5/1 -> Line buffer1/1, out_6/1
  Delay6/1 -> out_9/1
  Line buffer/1 -> Delay2/1, out_4/1
  Line buffer1/1 -> Delay3/1, out_7/1

== system gm_sobelFilter2024a/conv_core/sobel_horz_conv_core/Subsystem1/slicer ==
  channel_in : Inport  OutDataTypeStr=uint8  PortDimensions=1  SampleTime=2.77039007092199e-06
  Delay{1..6} (6 alike) : Delay  DelayLength=double(1)  InitialCondition=0
  Line buffer : Delay  DelayLength=double(750)  InitialCondition=0
  Line buffer1 : Delay  DelayLength=double(750)  InitialCondition=0
  out_1 : Outport  SampleTime=2.77039007092199e-06  InitialOutput=0  VectorParamsAs1DForOutWhenUnconnected=off
  out_2 : Outport  Port=2  SampleTime=2.77039007092199e-06  InitialOutput=0  VectorParamsAs1DForOutWhenUnconnected=off
  out_3 : Outport  Port=3  SampleTime=2.77039007092199e-06  InitialOutput=0  VectorParamsAs1DForOutWhenUnconnected=off
  out_4 : Outport  Port=4  SampleTime=2.77039007092199e-06  InitialOutput=0  VectorParamsAs1DForOutWhenUnconnected=off
  out_5 : Outport  Port=5  SampleTime=2.77039007092199e-06  InitialOutput=0  VectorParamsAs1DForOutWhenUnconnected=off
  out_6 : Outport  Port=6  SampleTime=2.77039007092199e-06  InitialOutput=0  VectorParamsAs1DForOutWhenUnconnected=off
  out_7 : Outport  Port=7  SampleTime=2.77039007092199e-06  InitialOutput=0  VectorParamsAs1DForOutWhenUnconnected=off
  out_8 : Outport  Port=8  SampleTime=2.77039007092199e-06  InitialOutput=0  VectorParamsAs1DForOutWhenUnconnected=off
  out_9 : Outport  Port=9  SampleTime=2.77039007092199e-06  InitialOutput=0  VectorParamsAs1DForOutWhenUnconnected=off
  wires:
  channel_in/1 -> Delay1/1, out_1/1
  Delay1/1 -> Delay4/1, out_2/1
  Delay2/1 -> Delay5/1, out_5/1
  Delay3/1 -> Delay6/1, out_8/1
  Delay4/1 -> Line buffer/1, out_3/1
  Delay5/1 -> Line buffer1/1, out_6/1
  Delay6/1 -> out_9/1
  Line buffer/1 -> Delay2/1, out_4/1
  Line buffer1/1 -> Delay3/1, out_7/1

== system gm_sobelFilter2024a/conv_core/sobel_horz_conv_core_alt/Subsystem1/slicer ==
  channel_in : Inport  OutDataTypeStr=uint8  PortDimensions=1  SampleTime=2.77039007092199e-06
  Delay{1..6} (6 alike) : Delay  DelayLength=double(1)  InitialCondition=0
  Line buffer : Delay  DelayLength=double(750)  InitialCondition=0
  Line buffer1 : Delay  DelayLength=double(750)  InitialCondition=0
  out_1 : Outport  SampleTime=2.77039007092199e-06  InitialOutput=0  VectorParamsAs1DForOutWhenUnconnected=off
  out_2 : Outport  Port=2  SampleTime=2.77039007092199e-06  InitialOutput=0  VectorParamsAs1DForOutWhenUnconnected=off
  out_3 : Outport  Port=3  SampleTime=2.77039007092199e-06  InitialOutput=0  VectorParamsAs1DForOutWhenUnconnected=off
  out_4 : Outport  Port=4  SampleTime=2.77039007092199e-06  InitialOutput=0  VectorParamsAs1DForOutWhenUnconnected=off
  out_5 : Outport  Port=5  SampleTime=2.77039007092199e-06  InitialOutput=0  VectorParamsAs1DForOutWhenUnconnected=off
  out_6 : Outport  Port=6  SampleTime=2.77039007092199e-06  InitialOutput=0  VectorParamsAs1DForOutWhenUnconnected=off
  out_7 : Outport  Port=7  SampleTime=2.77039007092199e-06  InitialOutput=0  VectorParamsAs1DForOutWhenUnconnected=off
  out_8 : Outport  Port=8  SampleTime=2.77039007092199e-06  InitialOutput=0  VectorParamsAs1DForOutWhenUnconnected=off
  out_9 : Outport  Port=9  SampleTime=2.77039007092199e-06  InitialOutput=0  VectorParamsAs1DForOutWhenUnconnected=off
  wires:
  channel_in/1 -> Delay1/1, out_1/1
  Delay1/1 -> Delay4/1, out_2/1
  Delay2/1 -> Delay5/1, out_5/1
  Delay3/1 -> Delay6/1, out_8/1
  Delay4/1 -> Line buffer/1, out_3/1
  Delay5/1 -> Line buffer1/1, out_6/1
  Delay6/1 -> out_9/1
  Line buffer/1 -> Delay2/1, out_4/1
  Line buffer1/1 -> Delay3/1, out_7/1

== system gm_sobelFilter2024a/conv_core/sobel_vert_conv_core/Subsystem1/slicer ==
  channel_in : Inport  OutDataTypeStr=uint8  PortDimensions=1  SampleTime=2.77039007092199e-06
  Delay{1..6} (6 alike) : Delay  DelayLength=double(1)  InitialCondition=0
  Line buffer : Delay  DelayLength=double(750)  InitialCondition=0
  Line buffer1 : Delay  DelayLength=double(750)  InitialCondition=0
  out_1 : Outport  SampleTime=2.77039007092199e-06  InitialOutput=0  VectorParamsAs1DForOutWhenUnconnected=off
  out_2 : Outport  Port=2  SampleTime=2.77039007092199e-06  InitialOutput=0  VectorParamsAs1DForOutWhenUnconnected=off
  out_3 : Outport  Port=3  SampleTime=2.77039007092199e-06  InitialOutput=0  VectorParamsAs1DForOutWhenUnconnected=off
  out_4 : Outport  Port=4  SampleTime=2.77039007092199e-06  InitialOutput=0  VectorParamsAs1DForOutWhenUnconnected=off
  out_5 : Outport  Port=5  SampleTime=2.77039007092199e-06  InitialOutput=0  VectorParamsAs1DForOutWhenUnconnected=off
  out_6 : Outport  Port=6  SampleTime=2.77039007092199e-06  InitialOutput=0  VectorParamsAs1DForOutWhenUnconnected=off
  out_7 : Outport  Port=7  SampleTime=2.77039007092199e-06  InitialOutput=0  VectorParamsAs1DForOutWhenUnconnected=off
  out_8 : Outport  Port=8  SampleTime=2.77039007092199e-06  InitialOutput=0  VectorParamsAs1DForOutWhenUnconnected=off
  out_9 : Outport  Port=9  SampleTime=2.77039007092199e-06  InitialOutput=0  VectorParamsAs1DForOutWhenUnconnected=off
  wires:
  channel_in/1 -> Delay1/1, out_1/1
  Delay1/1 -> Delay4/1, out_2/1
  Delay2/1 -> Delay5/1, out_5/1
  Delay3/1 -> Delay6/1, out_8/1
  Delay4/1 -> Line buffer/1, out_3/1
  Delay5/1 -> Line buffer1/1, out_6/1
  Delay6/1 -> out_9/1
  Line buffer/1 -> Delay2/1, out_4/1
  Line buffer1/1 -> Delay3/1, out_7/1

== system gm_sobelFilter2024a/conv_core/sobel_vert_conv_core_alt/Subsystem1/slicer ==
  channel_in : Inport  OutDataTypeStr=uint8  PortDimensions=1  SampleTime=2.77039007092199e-06
  Delay{1..6} (6 alike) : Delay  DelayLength=double(1)  InitialCondition=0
  Line buffer : Delay  DelayLength=double(750)  InitialCondition=0
  Line buffer1 : Delay  DelayLength=double(750)  InitialCondition=0
  out_1 : Outport  SampleTime=2.77039007092199e-06  InitialOutput=0  VectorParamsAs1DForOutWhenUnconnected=off
  out_2 : Outport  Port=2  SampleTime=2.77039007092199e-06  InitialOutput=0  VectorParamsAs1DForOutWhenUnconnected=off
  out_3 : Outport  Port=3  SampleTime=2.77039007092199e-06  InitialOutput=0  VectorParamsAs1DForOutWhenUnconnected=off
  out_4 : Outport  Port=4  SampleTime=2.77039007092199e-06  InitialOutput=0  VectorParamsAs1DForOutWhenUnconnected=off
  out_5 : Outport  Port=5  SampleTime=2.77039007092199e-06  InitialOutput=0  VectorParamsAs1DForOutWhenUnconnected=off
  out_6 : Outport  Port=6  SampleTime=2.77039007092199e-06  InitialOutput=0  VectorParamsAs1DForOutWhenUnconnected=off
  out_7 : Outport  Port=7  SampleTime=2.77039007092199e-06  InitialOutput=0  VectorParamsAs1DForOutWhenUnconnected=off
  out_8 : Outport  Port=8  SampleTime=2.77039007092199e-06  InitialOutput=0  VectorParamsAs1DForOutWhenUnconnected=off
  out_9 : Outport  Port=9  SampleTime=2.77039007092199e-06  InitialOutput=0  VectorParamsAs1DForOutWhenUnconnected=off
  wires:
  channel_in/1 -> Delay1/1, out_1/1
  Delay1/1 -> Delay4/1, out_2/1
  Delay2/1 -> Delay5/1, out_5/1
  Delay3/1 -> Delay6/1, out_8/1
  Delay4/1 -> Line buffer/1, out_3/1
  Delay5/1 -> Line buffer1/1, out_6/1
  Delay6/1 -> out_9/1
  Line buffer/1 -> Delay2/1, out_4/1
  Line buffer1/1 -> Delay3/1, out_7/1

== system gm_sobelFilter2024a/conv_core/sqrt_threshold/Subsystem2/slicer ==
  channel_in : Inport  OutDataTypeStr=uint8  PortDimensions=1  SampleTime=2.77039007092199e-06
  Delay1 : Delay  DelayLength=double(1)  InitialCondition=0
  Delay2 : Delay  DelayLength=double(1)  InitialCondition=0
  Delay4 : Delay  DelayLength=double(1)  InitialCondition=0
  Line buffer : Delay  DelayLength=double(750)  InitialCondition=0
  out_5 : Outport  SampleTime=2.77039007092199e-06  InitialOutput=0  VectorParamsAs1DForOutWhenUnconnected=off
  wires:
  channel_in/1 -> Delay1/1
  Delay1/1 -> Delay4/1
  Delay2/1 -> out_5/1
  Delay4/1 -> Line buffer/1
  Line buffer/1 -> Delay2/1

== system gm_sobelFilter2024a/conv_core/sqrt_threshold/Subsystem2/slicer1 ==
  channel_in : Inport  OutDataTypeStr=uint8  PortDimensions=1  SampleTime=2.77039007092199e-06
  Delay1 : Delay  DelayLength=double(1)  InitialCondition=0
  Delay2 : Delay  DelayLength=double(1)  InitialCondition=0
  Delay4 : Delay  DelayLength=double(1)  InitialCondition=0
  Line buffer : Delay  DelayLength=double(750)  InitialCondition=0
  out_5 : Outport  SampleTime=2.77039007092199e-06  InitialOutput=0  VectorParamsAs1DForOutWhenUnconnected=off
  wires:
  channel_in/1 -> Delay1/1
  Delay1/1 -> Delay4/1
  Delay2/1 -> out_5/1
  Delay4/1 -> Line buffer/1
  Line buffer/1 -> Delay2/1

== system gm_sobelFilter2024a/conv_core/sqrt_threshold1/Subsystem2/slicer ==
  channel_in : Inport  OutDataTypeStr=uint8  PortDimensions=1  SampleTime=2.77039007092199e-06
  Delay1 : Delay  DelayLength=double(1)  InitialCondition=0
  Delay2 : Delay  DelayLength=double(1)  InitialCondition=0
  Delay4 : Delay  DelayLength=double(1)  InitialCondition=0
  Line buffer : Delay  DelayLength=double(750)  InitialCondition=0
  out_5 : Outport  SampleTime=2.77039007092199e-06  InitialOutput=0  VectorParamsAs1DForOutWhenUnconnected=off
  wires:
  Line buffer/1 -> Delay2/1
  Delay4/1 -> Line buffer/1
  Delay2/1 -> out_5/1
  Delay1/1 -> Delay4/1
  channel_in/1 -> Delay1/1

== system gm_sobelFilter2024a/conv_core/sqrt_threshold1/Subsystem2/slicer1 ==
  channel_in : Inport  OutDataTypeStr=uint8  PortDimensions=1  SampleTime=2.77039007092199e-06
  Delay1 : Delay  DelayLength=double(1)  InitialCondition=0
  Delay2 : Delay  DelayLength=double(1)  InitialCondition=0
  Delay4 : Delay  DelayLength=double(1)  InitialCondition=0
  Line buffer : Delay  DelayLength=double(750)  InitialCondition=0
  out_5 : Outport  SampleTime=2.77039007092199e-06  InitialOutput=0  VectorParamsAs1DForOutWhenUnconnected=off
  wires:
  Line buffer/1 -> Delay2/1
  Delay4/1 -> Line buffer/1
  Delay2/1 -> out_5/1
  Delay1/1 -> Delay4/1
  channel_in/1 -> Delay1/1

== system gm_sobelFilter2024a/conv_core/sqrt_threshold2/Subsystem2/slicer ==
  channel_in : Inport  OutDataTypeStr=uint8  PortDimensions=1  SampleTime=2.77039007092199e-06
  Delay1 : Delay  DelayLength=double(1)  InitialCondition=0
  Delay2 : Delay  DelayLength=double(1)  InitialCondition=0
  Delay4 : Delay  DelayLength=double(1)  InitialCondition=0
  Line buffer : Delay  DelayLength=double(750)  InitialCondition=0
  out_5 : Outport  SampleTime=2.77039007092199e-06  InitialOutput=0  VectorParamsAs1DForOutWhenUnconnected=off
  wires:
  Line buffer/1 -> Delay2/1
  Delay4/1 -> Line buffer/1
  Delay2/1 -> out_5/1
  Delay1/1 -> Delay4/1
  channel_in/1 -> Delay1/1

== system gm_sobelFilter2024a/conv_core/sqrt_threshold2/Subsystem2/slicer1 ==
  channel_in : Inport  OutDataTypeStr=uint8  PortDimensions=1  SampleTime=2.77039007092199e-06
  Delay1 : Delay  DelayLength=double(1)  InitialCondition=0
  Delay2 : Delay  DelayLength=double(1)  InitialCondition=0
  Delay4 : Delay  DelayLength=double(1)  InitialCondition=0
  Line buffer : Delay  DelayLength=double(750)  InitialCondition=0
  out_5 : Outport  SampleTime=2.77039007092199e-06  InitialOutput=0  VectorParamsAs1DForOutWhenUnconnected=off
  wires:
  Line buffer/1 -> Delay2/1
  Delay4/1 -> Line buffer/1
  Delay2/1 -> out_5/1
  Delay1/1 -> Delay4/1
  channel_in/1 -> Delay1/1
